simulink model "Shema_9bus_sistem"  (R2023a)
settings: Solver=VariableStepAuto  StartTime=0.0  StopTime=10  RelTol=1e-3
libraries: spsThreePhaseVIMeasurementLib x9, spsLoadFlowBusLib x9, spsThreePhaseSeriesRLCBranchLib x6, spsFourierLib x3, spsMeanLib x3, spsPower3phInstantaneousLib x3, spsThreePhaseParallelRLCLoadLib x3, spsThreePhaseTransformerTwoWindingsLib x3, spsSynchronousMachinepuStandardLib x2, spsThreePhaseSourceLib x1, spspowerguiLib x1
settings Model: Creator=Ricardo Romero  LastModifiedBy=User
settings SolverCC: AlgebraicLoopSolver=TrustRegion
settings ModelReferenceCC: EnableRefExpFcnMdlSchedulingChecks=on

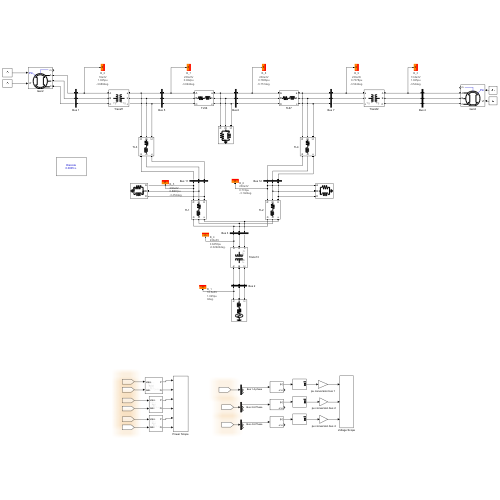
[thumbnail: Simulink's stored preview of the top-level diagram]
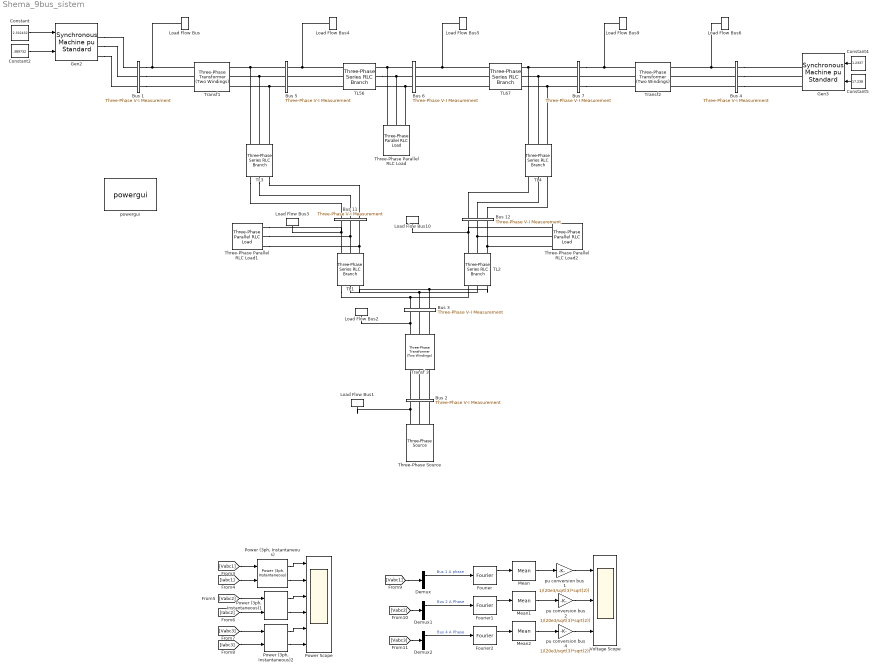
== system Shema_9bus_sistem ==
  Bus 1 : spsThreePhaseVIMeasurementLib/Three-Phase V-I Measurement  VoltageMeasurement=no  SetLabelV=on  LabelV=Vabc2  Vpu=off  VpuLL=off  CurrentMeasurement=no  SetLabelI=on  LabelI=Iabc2  Ipu=off  Pbase=100e6  Vbase=20e3  OutputType=Complex  PhasorSimulation=off  PSBequivalent=0
  Bus 11 : spsThreePhaseVIMeasurementLib/Three-Phase V-I Measurement  VoltageMeasurement=no  SetLabelV=on  LabelV=Vabc5  Vpu=off  VpuLL=off  CurrentMeasurement=no  SetLabelI=on  LabelI=Iabc5  Ipu=off  Pbase=100e6  Vbase=500e3  OutputType=Complex  PhasorSimulation=off  PSBequivalent=0
  Bus 12 : spsThreePhaseVIMeasurementLib/Three-Phase V-I Measurement  VoltageMeasurement=no  SetLabelV=on  LabelV=Vabc6  Vpu=off  VpuLL=off  CurrentMeasurement=no  SetLabelI=on  LabelI=Iabc6  Ipu=off  Pbase=100e6  Vbase=500e3  OutputType=Complex  PhasorSimulation=off  PSBequivalent=0
  Bus 2 : spsThreePhaseVIMeasurementLib/Three-Phase V-I Measurement  VoltageMeasurement=no  SetLabelV=on  LabelV=Vabc1  Vpu=off  VpuLL=off  CurrentMeasurement=no  SetLabelI=on  LabelI=Iabc1  Ipu=off  Pbase=100e6  Vbase=20e3  OutputType=Complex  PhasorSimulation=off  PSBequivalent=0
  Bus 3 : spsThreePhaseVIMeasurementLib/Three-Phase V-I Measurement  VoltageMeasurement=no  SetLabelV=on  LabelV=Vabc4  Vpu=off  VpuLL=off  CurrentMeasurement=no  SetLabelI=on  LabelI=Iabc4  Ipu=off  Pbase=100e6  Vbase=500e3  OutputType=Complex  PhasorSimulation=off  PSBequivalent=0
  Bus 4 : spsThreePhaseVIMeasurementLib/Three-Phase V-I Measurement  VoltageMeasurement=no  SetLabelV=on  LabelV=Vabc3  Vpu=off  VpuLL=off  CurrentMeasurement=no  SetLabelI=on  LabelI=Iabc3  Ipu=off  Pbase=100e6  Vbase=20e3  OutputType=Complex  PhasorSimulation=off  PSBequivalent=0
  Bus 5 : spsThreePhaseVIMeasurementLib/Three-Phase V-I Measurement  VoltageMeasurement=no  SetLabelV=on  LabelV=Vabc7  Vpu=off  VpuLL=off  CurrentMeasurement=no  SetLabelI=on  LabelI=Iabc7  Ipu=off  Pbase=100e6  Vbase=500e3  OutputType=Complex  PhasorSimulation=off  PSBequivalent=0
  Bus 6 : spsThreePhaseVIMeasurementLib/Three-Phase V-I Measurement  VoltageMeasurement=no  SetLabelV=on  LabelV=Vabc8  Vpu=off  VpuLL=off  CurrentMeasurement=no  SetLabelI=on  LabelI=Iabc8  Ipu=off  Pbase=100e6  Vbase=500e3  OutputType=Complex  PhasorSimulation=off  PSBequivalent=0
  Bus 7 : spsThreePhaseVIMeasurementLib/Three-Phase V-I Measurement  VoltageMeasurement=no  SetLabelV=on  LabelV=Vabc9  Vpu=off  VpuLL=off  CurrentMeasurement=no  SetLabelI=on  LabelI=Iabc9  Ipu=off  Pbase=100e6  Vbase=500e3  OutputType=Complex  PhasorSimulation=off  PSBequivalent=0
  Constant : Constant  Value=2.332432
  Constant2 : Constant  Value=.389732
  Constant4 : Constant  Value=1.2337
  Constant5 : Constant  Value=17.238
  Demux : Demux  Outputs=3
  Demux1 : Demux  Outputs=3
  Demux2 : Demux  Outputs=3
  Fourier : spsFourierLib/Fourier  Freq=60  n=1  InInit=[0, 0]  Ts=0
  Fourier1 : spsFourierLib/Fourier  Freq=60  n=1  InInit=[0, 0]  Ts=0
  Fourier2 : spsFourierLib/Fourier  Freq=60  n=1  InInit=[0, 0]  Ts=0
  Gen2 : spsSynchronousMachinepuStandardLib/Synchronous Machine pu Standard  PresetModel=No  MechanicalLoad=Mechanical power Pm  ShowDetailedParameters=on  RotorType=Round  Units=per unit standard parameters  MeasurementBus=off  NominalParameters=[163e6 18e3 60]  Reactances1=[0.8958 .1198 .25 1.7 .8645 .1969 .220]  Reactances2=[2.24 0.17 0.12 1.02 0.13 0.08]  dAxisTimeConstants=Open-circuit  qAxisTimeConstants=Open-circuit  TimeConstants1="[ 4.4849  0.0681  0.1  ]"  TimeConstants2=[6 .03 .535 .05]  TimeConstants3="[  4.49  0.0681  0.0513  ]"  TimeConstants4=[ 8.0, 0.03, 0.3371, 0.0295 ]  TimeConstants5=[ 1.01, 0.053, 0.1 ]  TimeConstants6=[ 1.3201, 0.023, 1.0, 0.07 ]  TimeConstants7=[0.012 0.003 0.003]  TimeConstants8=[ 1.3201, 0.0231, 0.3371, 0.0295 ]  StatorResistance=0.0025  Mechanical="[ 6.4  0  4]"  PolePairs=20  InitialConditions=[0 -49.7606 0.508854 0.508854 0.508854 0.2685 -119.731 120.269 1.07624]  SetSaturation=off  Saturation=[0.6404,0.7127,0.8441,0.9214,0.9956,1.082,1.19,1.316,1.457;0.7,0.7698,0.8872,0.9466,0.9969,1.046,1.1,1.151,1.201]  LoadFlowParameters=[1,0,0,0,0]  TsPowergui=0  TsBlock=-1  IterativeModel=Trapezoidal non iterative  IterativeDiscreteModel=Trapezoidal non iterative  BusType=PV  Pref=163000000  Qref=185000000  Qmin=-Inf  Qmax=Inf  PLF=0  QLF=0
  Gen3 : spsSynchronousMachinepuStandardLib/Synchronous Machine pu Standard  PresetModel=No  MechanicalLoad=Mechanical power Pm  ShowDetailedParameters=on  RotorType=Round  Units=per unit standard parameters  MeasurementBus=off  NominalParameters=[85e6 13.8e3 60]  Reactances1=[1.3125 .1813 .25 1.2578 .25 .25 .246]  Reactances2=[2.24 0.17 0.12 1.02 0.13 0.08]  dAxisTimeConstants=Open-circuit  qAxisTimeConstants=Open-circuit  TimeConstants1="[ 4.4849  0.0681  0.1  ]"  TimeConstants2=[5.89 .03 .6 .05]  TimeConstants3="[  4.49  0.0681  0.0513  ]"  TimeConstants4=[ 8.0, 0.03, 0.3371, 0.0295 ]  TimeConstants5=[ 1.01, 0.053, 0.1 ]  TimeConstants6=[ 1.3201, 0.023, 1.0, 0.07 ]  TimeConstants7=[0.012 0.003 0.003]  TimeConstants8=[ 1.3201, 0.0231, 0.3371, 0.0295 ]  StatorResistance=0.0025  Mechanical="[ 3.01  0  4]"  PolePairs=20  InitialConditions=[0 -46.9087 0.68512 0.68512 0.68512 7.5546 -112.445 127.555 1.27256]  SetSaturation=off  Saturation=[0.6404,0.7127,0.8441,0.9214,0.9956,1.082,1.19,1.316,1.457;0.7,0.7698,0.8872,0.9466,0.9969,1.046,1.1,1.151,1.201]  LoadFlowParameters=[1,0,0,0,0]  TsPowergui=0  TsBlock=-1  IterativeModel=Trapezoidal non iterative  IterativeDiscreteModel=Trapezoidal non iterative  BusType=PV  Pref=83000000  Qref=202000000  Qmin=-Inf  Qmax=Inf  PLF=0  QLF=0
  Load Flow Bus : spsLoadFlowBusLib/Load Flow Bus  LConnTagsString=a  Phases=single  Connectors=on one side  ID=B_2  Vbase=18e3  Vref=1.025  Vangle=0  VLF=1.025  VLFb=1  VLFc=1  angleLF=-3.689  angleLFb=0  angleLFc=0
  Load Flow Bus1 : spsLoadFlowBusLib/Load Flow Bus  LConnTagsString=a  Phases=single  Connectors=on one side  ID=B_1  Vbase=16.5e3  Vref=1.04  Vangle=0  VLF=1.025  VLFb=1  VLFc=1  angleLF=0  angleLFb=0  angleLFc=0
  Load Flow Bus10 : spsLoadFlowBusLib/Load Flow Bus  LConnTagsString=a  Phases=single  Connectors=on one side  ID=B_6  Vbase=230e3  Vref=1  Vangle=0  VLF=0.774  VLFb=1  VLFc=1  angleLF=-3.142  angleLFb=0  angleLFc=0
  Load Flow Bus2 : spsLoadFlowBusLib/Load Flow Bus  LConnTagsString=a  Phases=single  Connectors=on one side  ID=B_4  Vbase=230e3  Vref=1  Vangle=0  VLF=0.8455  VLFb=1  VLFc=1  angleLF=-0.02924  angleLFb=0  angleLFc=0
  Load Flow Bus3 : spsLoadFlowBusLib/Load Flow Bus  LConnTagsString=a  Phases=single  Connectors=on one side  ID=B_5  Vbase=230e3  Vref=1  Vangle=0  VLF=0.8807  VLFb=1  VLFc=1  angleLF=-3.452  angleLFb=0  angleLFc=0
  Load Flow Bus4 : spsLoadFlowBusLib/Load Flow Bus  LConnTagsString=a  Phases=single  Connectors=on one side  ID=B_7  Vbase=230e3  Vref=1  Vangle=0  VLF=0.922  VLFb=1  VLFc=1  angleLF=-3.694  angleLFb=0  angleLFc=0
  Load Flow Bus5 : spsLoadFlowBusLib/Load Flow Bus  LConnTagsString=a  Phases=single  Connectors=on one side  ID=B_8  Vbase=230e3  Vref=1  Vangle=0  VLF=0.7656  VLFb=1  VLFc=1  angleLF=-5.751  angleLFb=0  angleLFc=0
  Load Flow Bus6 : spsLoadFlowBusLib/Load Flow Bus  LConnTagsString=a  Phases=single  Connectors=on one side  ID=B_3  Vbase=13.8e3  Vref=1.025  Vangle=0  VLF=1.025  VLFb=1  VLFc=1  angleLF=-3.54  angleLFb=0  angleLFc=0
  Load Flow Bus9 : spsLoadFlowBusLib/Load Flow Bus  LConnTagsString=a  Phases=single  Connectors=on one side  ID=B_9  Vbase=230e3  Vref=1  Vangle=0  VLF=0.7078  VLFb=1  VLFc=1  angleLF=-3.544  angleLFb=0  angleLFc=0
  Mean : spsMeanLib/Mean  Freq=60  Vinit=0  Ts=0
  Mean1 : spsMeanLib/Mean  Freq=60  Vinit=0  Ts=0
  Mean2 : spsMeanLib/Mean  Freq=60  Vinit=0  Ts=0
  "Power (3ph, Instantaneous)" : spsPower3phInstantaneousLib/Power (3ph, Instantaneous)
  "Power (3ph, Instantaneous)1" : spsPower3phInstantaneousLib/Power (3ph, Instantaneous)
  "Power (3ph, Instantaneous)2" : spsPower3phInstantaneousLib/Power (3ph, Instantaneous)
  Power Scope : Scope  NumInputPorts=6
  TL1 : spsThreePhaseSeriesRLCBranchLib/Three-Phase Series RLC Branch  LConnTagsString=A|B|C  RConnTagsString=A|B|C  BranchType=RL  Resistance=0.529  Inductance=1.403e-2  Capacitance=1e-6  Measurements=None
  TL2 : spsThreePhaseSeriesRLCBranchLib/Three-Phase Series RLC Branch  LConnTagsString=A|B|C  RConnTagsString=A|B|C  BranchType=RL  Resistance=0.529  Inductance=1.403e-2  Capacitance=1e-6  Measurements=None
  TL3 : spsThreePhaseSeriesRLCBranchLib/Three-Phase Series RLC Branch  LConnTagsString=A|B|C  RConnTagsString=A|B|C  BranchType=RL  Resistance=0.032  Inductance=0.161/(2*pi*60)  Capacitance=1e-6  Measurements=None
  TL4 : spsThreePhaseSeriesRLCBranchLib/Three-Phase Series RLC Branch  LConnTagsString=A|B|C  RConnTagsString=A|B|C  BranchType=RL  Resistance=0.039  Inductance=0.17/(2*pi*60)  Capacitance=1e-6  Measurements=None
  TL56 : spsThreePhaseSeriesRLCBranchLib/Three-Phase Series RLC Branch  LConnTagsString=A|B|C  RConnTagsString=A|B|C  BranchType=RL  Resistance=0.0085  Inductance=0.072/(2*pi*60)  Capacitance=1e-6  Measurements=None
  TL67 : spsThreePhaseSeriesRLCBranchLib/Three-Phase Series RLC Branch  LConnTagsString=A|B|C  RConnTagsString=A|B|C  BranchType=RL  Resistance=0.0119  Inductance=0.1008/(2*pi*60)  Capacitance=1e-6  Measurements=None
  Three-Phase Parallel RLC Load : spsThreePhaseParallelRLCLoadLib/Three-Phase Parallel RLC Load  LConnTagsString=A|B|C  Configuration=Y (grounded)  NominalVoltage=(230000)*1.01675  Vabc=[1e3 1e3 1e3]  Vabcp=[1e3 1e3 1e3]  NominalFrequency=60  UnbalancedPower=off  ActivePower=100e6  InductivePower=35e6  CapacitivePower=0  Pabc=[10e3 9e3 11e3]  QLabc=[100 90 110]  QCabc=[100 90 110]  Pabcp=[10e3 9e3 11e3]  QLabcp=[100 90 110]  QCabcp=[100 90 110]  Measurements=None  LoadType=constant PQ
  Three-Phase Parallel RLC Load1 : spsThreePhaseParallelRLCLoadLib/Three-Phase Parallel RLC Load  LConnTagsString=A|B|C  Configuration=Y (grounded)  NominalVoltage=(230000)*1.01675  Vabc=[1e3 1e3 1e3]  Vabcp=[1e3 1e3 1e3]  NominalFrequency=60  UnbalancedPower=off  ActivePower=125e6  InductivePower=50e6  CapacitivePower=0  Pabc=[10e3 9e3 11e3]  QLabc=[100 90 110]  QCabc=[100 90 110]  Pabcp=[10e3 9e3 11e3]  QLabcp=[100 90 110]  QCabcp=[100 90 110]  Measurements=None  LoadType=constant PQ
  Three-Phase Parallel RLC Load2 : spsThreePhaseParallelRLCLoadLib/Three-Phase Parallel RLC Load  LConnTagsString=A|B|C  Configuration=Y (grounded)  NominalVoltage=(230000)*1.01675  Vabc=[1e3 1e3 1e3]  Vabcp=[1e3 1e3 1e3]  NominalFrequency=60  UnbalancedPower=off  ActivePower=90e6  InductivePower=30e5  CapacitivePower=0  Pabc=[10e3 9e3 11e3]  QLabc=[100 90 110]  QCabc=[100 90 110]  Pabcp=[10e3 9e3 11e3]  QLabcp=[100 90 110]  QCabcp=[100 90 110]  Measurements=None  LoadType=constant PQ
  Three-Phase Source : spsThreePhaseSourceLib/Three-Phase Source  InternalConnection=Yg  VoltagePhases=off  Voltage=16.5e3  PhaseAngle=0  Voltage_phases=[25e3 25e3 25e3]/sqrt(3)  PhaseAngles_phases=[0 -120 +120]  Frequency=60  NonIdealSource=on  SpecifyImpedance=off  Resistance=0.8929  Inductance=16.58e-3  ShortCircuitLevel=100e6  BaseVoltage=16.5e3  XRratio=7  BusType=swing  Pref=10e3  Qref=0  Prefabc=[10e3, 10e3, 10e3]  Qrefabc=[0, 0, 0]  Qmin=-inf  Qmax=inf
  Transf 3 : spsThreePhaseTransformerTwoWindingsLib/Three-Phase Transformer (Two Windings)  Winding1Connection=Yg  Winding2Connection=Yg  CoreType=Three single-phase transformers  SetSaturation=off  Hysteresis=off  DataFile='hysteresis'  SetInitialFlux=off  Measurements=None  UNITS=pu  NominalPower=[ 100e6 , 60 ]  Winding1=[ 16.5e3 , 1e-6, 0.0576/(2*3.14*60*2) ]  Winding2=[ 230e3 ,1e-6, 0.0576/(2*3.14*60*2) ]  Rm=500  Lm=500  L0=0.5  Saturation=[0 0;0.0024 1.2;0.99999 1.52]  InitialFluxes=[ 0.8 , -0.8 , 0.7 ]  BreakLoop=off  DiscreteSolver=Trapezoidal iterative  DataType=off  TransfoNumber=1
  Transf1 : spsThreePhaseTransformerTwoWindingsLib/Three-Phase Transformer (Two Windings)  Winding1Connection=Yg  Winding2Connection=Yg  CoreType=Three single-phase transformers  SetSaturation=off  Hysteresis=off  DataFile='hysteresis'  SetInitialFlux=off  Measurements=None  UNITS=pu  NominalPower=[100e6,60]  Winding1=[ 18e3 , 1e-6 , 0.0625/(2*3.14*60*2)]  Winding2=[ 230e3 , 1e-6, 0.0625/(2*3.14*60*2) ]  Rm=500  Lm=500  L0=0.5  Saturation=[0 0;0.0024001 1.2;0.99998 1.52]  InitialFluxes=[ 0.8 , -0.8 , 0.7 ]  BreakLoop=off  DiscreteSolver=Trapezoidal iterative  DataType=off  TransfoNumber=1
  Transf2 : spsThreePhaseTransformerTwoWindingsLib/Three-Phase Transformer (Two Windings)  Winding1Connection=Yg  Winding2Connection=Yg  CoreType=Three single-phase transformers  SetSaturation=off  Hysteresis=off  DataFile='hysteresis'  SetInitialFlux=off  Measurements=None  UNITS=pu  NominalPower=[100e6,60]  Winding1=[ 13.8e3 , 1e-6 , 0.0586/(2*3.14*60*2) ]  Winding2=[ 230e3 , 1e-6, 0.0586/(2*3.14*60*2) ]  Rm=500  Lm=500  L0=0.5  Saturation=[0 0;0.0024 1.2;0.99999 1.52]  InitialFluxes=[ 0.8 , -0.8 , 0.7 ]  BreakLoop=off  DiscreteSolver=Trapezoidal iterative  DataType=off  TransfoNumber=1
  Voltage Scope : Scope  NumInputPorts=3
  powergui : spspowerguiLib/powergui  Priority=1  SimulationMode=Discrete  SampleTime=500e-6  frequency=60  Iterations=50  frequencyindice=60  Pbase=100e6  ErrMax=0.0001  UnitsV=kV  UnitsW=MW  buscounter=2  FunctionMessages=off  echomessages=off  EnableUseOfTLC=off  CurrentSourceSwitches=off  DisableSnubberDevices=off  DisableRonSwitches=off  DisableVfSwitches=off  DisplayEquations=off  AutomaticDiscreteSolvers=on  SolverType=Tustin/Backward Euler (TBE)  Interpol=off  ExternalGateDelay=off  methode=off  Ts=100  x0status=blocks  SPID=on  SwTol=0  HookPort=off  NonlinearTolerance=1e-4  nMaxIteration=100  ContinueOnMaxIteration=off  RestoreLinks=warning  ResistiveCurrentMeasurement=off  Frange=[0:2:500]  Ylog=off  Xlog=on  ShowGrid=off  save=off  variable=ZData  structure=0  ZoomFFT=off  StartTime=0.0  cycles=1  DisplayStyle=1  fundamental=60  FreqAxis=off  MaxFrequency=1000  frequencyindicesteady=1  RmsSteady=1  display=off
  pu conversion bus 1 : Gain  Gain=1/(20e3/sqrt(3)*sqrt(2))
  pu conversion bus 2 : Gain  Gain=1/(20e3/sqrt(3)*sqrt(2))
  pu conversion bus 4 : Gain  Gain=1/(20e3/sqrt(3)*sqrt(2))
  wires:
  [Vabc1] -> "Power (3ph, Instantaneous)"/1
  [Iabc1] -> "Power (3ph, Instantaneous)"/2
  "Power (3ph, Instantaneous)"/1 -> Power Scope/1
  "Power (3ph, Instantaneous)"/2 -> Power Scope/2
  [Vabc2] -> "Power (3ph, Instantaneous)1"/1
  [Iabc2] -> "Power (3ph, Instantaneous)1"/2
  [Vabc3] -> "Power (3ph, Instantaneous)2"/1
  [Iabc3] -> "Power (3ph, Instantaneous)2"/2
  "Power (3ph, Instantaneous)2"/2 -> Power Scope/6
  "Power (3ph, Instantaneous)2"/1 -> Power Scope/5
  "Power (3ph, Instantaneous)1"/2 -> Power Scope/4
  "Power (3ph, Instantaneous)1"/1 -> Power Scope/3
  [Vabc1] -> Demux/1
  Demux/1 -> Fourier/1  "Bus 1 A phase"
  Demux1/1 -> Fourier1/1  "Bus 2 A Phase"
  [Vabc2] -> Demux1/1
  Demux2/1 -> Fourier2/1  "Bus 4 A Phase"
  [Vabc3] -> Demux2/1
  pu conversion bus 1/1 -> Voltage Scope/1
  pu conversion bus 2/1 -> Voltage Scope/2
  pu conversion bus 4/1 -> Voltage Scope/3
  Fourier/1 -> Mean/1
  Mean/1 -> pu conversion bus 1/1
  Fourier1/1 -> Mean1/1
  Mean1/1 -> pu conversion bus 2/1
  Mean2/1 -> pu conversion bus 4/1
  Fourier2/1 -> Mean2/1
  Constant/1 -> Gen2/1
  Constant2/1 -> Gen2/2
  Constant4/1 -> Gen3/1
  Constant5/1 -> Gen3/2
  connections:
  Gen2/RConn1 -- Bus 1/LConn1
  Gen2/RConn2 -- Bus 1/LConn2
  Gen2/RConn3 -- Bus 1/LConn3
  Bus 1/RConn1 -- Load Flow Bus/LConn1 -- Transf1/LConn1
  Bus 1/RConn2 -- Transf1/LConn2
  Bus 1/RConn3 -- Transf1/LConn3
  Bus 5/LConn1 -- TL3/LConn1 -- Transf1/RConn1
  Bus 5/LConn2 -- TL3/LConn2 -- Transf1/RConn2
  Bus 5/LConn3 -- TL3/LConn3 -- Transf1/RConn3
  Bus 6/LConn1 -- Three-Phase Parallel RLC Load/LConn1 -- TL56/RConn1
  Bus 6/LConn3 -- Three-Phase Parallel RLC Load/LConn3 -- TL56/RConn3
  TL56/LConn1 -- Load Flow Bus4/LConn1 -- Bus 5/RConn1
  TL56/LConn2 -- Bus 5/RConn2
  TL56/LConn3 -- Bus 5/RConn3
  TL67/LConn1 -- Load Flow Bus5/LConn1 -- Bus 6/RConn1
  TL67/LConn2 -- Bus 6/RConn2
  TL67/LConn3 -- Bus 6/RConn3
  Bus 7/LConn1 -- TL4/LConn1 -- TL67/RConn1
  Bus 7/LConn2 -- TL4/LConn2 -- TL67/RConn2
  Bus 7/LConn3 -- TL4/LConn3 -- TL67/RConn3
  Load Flow Bus9/LConn1 -- Transf2/RConn1 -- Bus 7/RConn1
  Transf2/RConn2 -- Bus 7/RConn2
  Bus 7/RConn3 -- Transf2/RConn3
  Bus 2/RConn1 -- Transf 3/LConn1
  Bus 2/RConn2 -- Transf 3/LConn2
  Bus 2/RConn3 -- Transf 3/LConn3
  TL56/RConn2 -- Three-Phase Parallel RLC Load/LConn2 -- Bus 6/LConn2
  Bus 4/LConn1 -- Load Flow Bus6/LConn1 -- Transf2/LConn1
  Bus 4/LConn2 -- Transf2/LConn2
  Bus 4/LConn3 -- Transf2/LConn3
  Bus 4/RConn1 -- Gen3/RConn1
  Bus 4/RConn2 -- Gen3/RConn2
  Bus 4/RConn3 -- Gen3/RConn3
  Transf 3/RConn1 -- Load Flow Bus2/LConn1 -- Bus 3/RConn3
  Transf 3/RConn2 -- Bus 3/RConn2
  Transf 3/RConn3 -- Bus 3/RConn1
  TL1/RConn1 -- TL2/RConn1 -- Bus 3/LConn3
  TL1/RConn2 -- TL2/RConn2 -- Bus 3/LConn2
  TL1/RConn3 -- TL2/RConn3 -- Bus 3/LConn1
  TL1/LConn1 -- Three-Phase Parallel RLC Load1/LConn1 -- Bus 11/RConn3 -- Load Flow Bus3/LConn1
  TL1/LConn2 -- Three-Phase Parallel RLC Load1/LConn2 -- Bus 11/RConn2
  TL1/LConn3 -- Three-Phase Parallel RLC Load1/LConn3 -- Bus 11/RConn1
  TL2/LConn1 -- Three-Phase Parallel RLC Load2/LConn1 -- Bus 12/RConn3 -- Load Flow Bus10/LConn1
  TL2/LConn2 -- Three-Phase Parallel RLC Load2/LConn2 -- Bus 12/RConn2
  TL2/LConn3 -- Three-Phase Parallel RLC Load2/LConn3 -- Bus 12/RConn1
  TL3/RConn1 -- Bus 11/LConn3
  TL3/RConn2 -- Bus 11/LConn2
  TL3/RConn3 -- Bus 11/LConn1
  Bus 12/LConn3 -- TL4/RConn1
  Bus 12/LConn2 -- TL4/RConn2
  Bus 12/LConn1 -- TL4/RConn3
  Load Flow Bus1/LConn1 -- Three-Phase Source/RConn1 -- Bus 2/LConn1
  Three-Phase Source/RConn2 -- Bus 2/LConn2
  Three-Phase Source/RConn3 -- Bus 2/LConn3
